simulink model "two_level_sixphase_f_sw_counter"  (R2021a)
settings: Solver=FixedStepDiscrete  StartTime=0.0  StopTime=0.030  RelTol=1e-3
libraries: hdlsllib x1
settings Model: DataTypeOverride=Off  Creator=micha  LastModifiedBy=micha
settings SolverCC: AlgebraicLoopSolver=TrustRegion  AutoInsertRateTranBlk=on
settings DataIOCC: LimitDataPoints=on  SaveOutput=off  SaveTime=off
settings OptimizationCC: BlockReduction=off  ConditionallyExecuteInputs=off  DefaultParameterBehavior=Inlined  LifeSpan=inf
settings DebuggingCC: AlgebraicLoopMsg=error  SingleTaskRateTransMsg=error  AllowSymbolicDim=off  StrictBusMsg=ErrorOnBusTreatedAsVector  SFUnexpectedBacktrackingDiag=warning  SFNoUnconditionalDefaultTransitionDiag=warning  SFExecutionAtInitializationDiag=none  SFMachineParentedDataDiag=warning  ArithmeticOperatorsInVariantConditions=warning
settings HardwareCC: ProdBitPerPointer=32  ProdBitPerSizeT=32  ProdBitPerPtrDiffT=32  ProdLargestAtomicFloat=None  ProdIntDivRoundTo=Undefined  ProdEndianess=Unspecified  ProdWordSize=32  ProdHWDeviceType=ASIC/FPGA->ASIC/FPGA  ProdEqTarget=off
settings SFSimCC: SimUseLocalCustomCode=off  CustomCodeUndefinedFunction=UseInterfaceOnly
settings RTWCC: RTWUseLocalCustomCode=off
settings CodeAppCC: StateflowObjectComments=on
settings GRTTargetCC: TargetLangStandard=C89/C90 (ANSI)
settings ConfigComp: CovScope=ReferencedModels  CovMetricSettings=dw  CovSaveCumulativeToWorkspaceVar=on  CovSaveSingleToWorkspaceVar=on  CovExternalEMLEnable=off  CovSFcnEnable=off

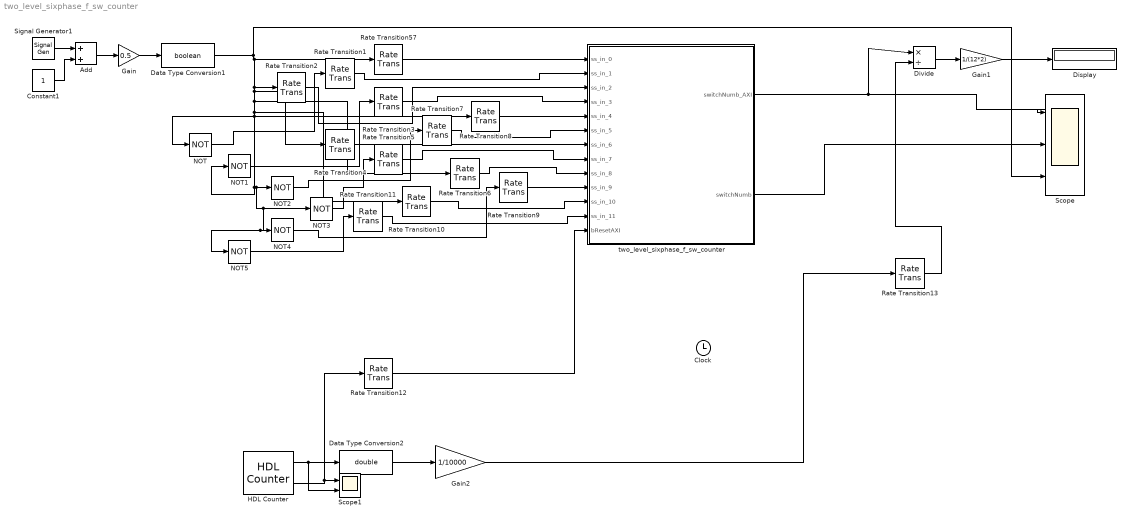
== system two_level_sixphase_f_sw_counter ==
  Add : Sum
  Clock : Clock
  Constant1 : Constant
  Data Type Conversion1 : DataTypeConversion  OutDataTypeStr=boolean
  Data Type Conversion2 : DataTypeConversion  OutDataTypeStr=double
  Display : Display
  Divide : Product  Inputs=*/
  Gain : Gain  Gain=0.5
  Gain1 : Gain  Gain=1/(12*2)
  Gain2 : Gain  Gain=1/10000
  HDL Counter : hdlsllib/Sources/HDL Counter  CountType=Count limited  CountInit=0  CountStep=1  CountMax=100  CountFromType=Initial value  CountFrom=0  CountResetPort=off  CountLoadPort=off  CountEnbPort=off  CountDirPort=off  CountHitOutputPort=on  CountDataType=Unsigned  CountWordLen=32  CountFracLen=0  CountSampTime=100e-6
  NOT{,1..5} (6 alike) : Logic  Operator=NOT  IconShape=distinctive  AllPortsSameDT=off  OutDataTypeStr=boolean
  Rate Transition{1..13,57} (14 alike) : RateTransition  OutPortSampleTime=t_clock
  Scope : Scope  NumInputPorts=3
  Scope1 : Scope  NumInputPorts=2
  Signal Generator1 : SignalGenerator  WaveForm=square  Frequency=2*pi*10000  Units=rad/sec
  two_level_sixphase_f_sw_counter : Subsystem  TreatAsAtomicUnit=on
  wires:
  Rate Transition57/1 -> two_level_sixphase_f_sw_counter/1(ss_in_0)
  Rate Transition1/1 -> two_level_sixphase_f_sw_counter/2(ss_in_1)
  Rate Transition2/1 -> two_level_sixphase_f_sw_counter/3(ss_in_2)
  Rate Transition3/1 -> two_level_sixphase_f_sw_counter/4(ss_in_3)
  Rate Transition4/1 -> two_level_sixphase_f_sw_counter/7(ss_in_6)
  Rate Transition5/1 -> two_level_sixphase_f_sw_counter/8(ss_in_7)
  Rate Transition6/1 -> two_level_sixphase_f_sw_counter/9(ss_in_8)
  Rate Transition7/1 -> two_level_sixphase_f_sw_counter/6(ss_in_5)
  Rate Transition8/1 -> two_level_sixphase_f_sw_counter/5(ss_in_4)
  Rate Transition9/1 -> two_level_sixphase_f_sw_counter/10(ss_in_9)
  Rate Transition10/1 -> two_level_sixphase_f_sw_counter/11(ss_in_10)
  Rate Transition11/1 -> two_level_sixphase_f_sw_counter/12(ss_in_11)
  HDL Counter/2 -> Scope1/1, Rate Transition12/1
  Rate Transition12/1 -> two_level_sixphase_f_sw_counter/13(bResetAXI)
  two_level_sixphase_f_sw_counter/1(switchNumb_AXI) -> Scope/1, Divide/1
  two_level_sixphase_f_sw_counter/2(switchNumb) -> Scope/2
  Add/1 -> Gain/1
  Signal Generator1/1 -> Add/1
  Constant1/1 -> Add/2
  Gain/1 -> Data Type Conversion1/1
  Data Type Conversion1/1 -> Rate Transition57/1, Rate Transition4/1, Rate Transition6/1, Rate Transition10/1, NOT5/1, NOT4/1, NOT3/1, NOT2/1, NOT1/1, NOT/1, Rate Transition8/1, Rate Transition2/1, Scope/3
  NOT/1 -> Rate Transition1/1
  NOT1/1 -> Rate Transition3/1
  NOT2/1 -> Rate Transition7/1
  NOT3/1 -> Rate Transition5/1
  NOT4/1 -> Rate Transition9/1
  NOT5/1 -> Rate Transition11/1
  Divide/1 -> Gain1/1
  Gain1/1 -> Display/1
  HDL Counter/1 -> Data Type Conversion2/1, Scope1/2
  Rate Transition13/1 -> Divide/2
  Gain2/1 -> Rate Transition13/1
  Data Type Conversion2/1 -> Gain2/1

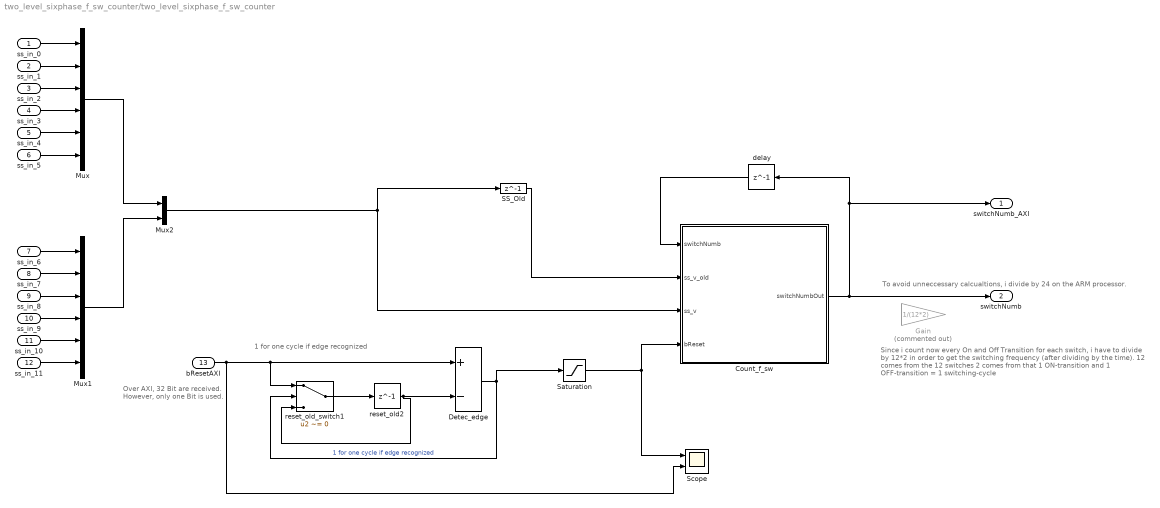
== system two_level_sixphase_f_sw_counter/two_level_sixphase_f_sw_counter ==
  note: To avoid unneccessary calcualtions, i divide by 24 on the ARM processor.
  note: 1 for one cycle if edge recognized
  note: Over AXI, 32 Bit are received.
      | However, only one Bit is used.
  note: Since i count now every On and Off Transition for each switch,
      |  i have to divide by 12*2 in order to get the switching frequency
      |  (after dividing by the time).
      | 12 comes from the 12 switches
      | 2 comes from that 1 ON-transition and 1 OFF-transition = 1 switching-cycle
  ss_in_0 : Inport
  ss_in_1 : Inport  Port=2
  ss_in_2 : Inport  Port=3
  ss_in_3 : Inport  Port=4
  ss_in_4 : Inport  Port=5
  ss_in_5 : Inport  Port=6
  ss_in_6 : Inport  Port=7
  ss_in_7 : Inport  Port=8
  ss_in_8 : Inport  Port=9
  ss_in_9 : Inport  Port=10
  ss_in_10 : Inport  Port=11
  ss_in_11 : Inport  Port=12
  bResetAXI : Inport  Port=13
  Count_f_sw : MATLAB Function  TreatAsAtomicUnit=on  VariantControl=(default)
  Detec_edge : Sum  Inputs=+-  AccumDataTypeStr=int8  OutDataTypeStr=int8
  Gain : Gain  Commented=on  Gain=1/(12*2)
  Mux : Mux  Inputs=6
  Mux1 : Mux  Inputs=6
  Mux2 : Mux  Inputs=2
  SS_Old : Delay  DelayLength=1
  Saturation : Saturate  UpperLimit=1  LowerLimit=0  OutMin=[0]  OutMax=[1]  OutDataTypeStr=fixdt(0,1)
  Scope : Scope  NumInputPorts=2
  delay : Delay  DelayLength=1
  reset_old2 : Delay  DelayLength=1
  reset_old_switch1 : Switch  Criteria=u2 ~= 0
  switchNumb_AXI : Outport  VectorParamsAs1DForOutWhenUnconnected=off
  switchNumb : Outport  Port=2  VectorParamsAs1DForOutWhenUnconnected=off
  wires:
  Count_f_sw/1(switchNumbOut) -> delay/1, switchNumb_AXI/1, switchNumb/1
  SS_Old/1 -> Count_f_sw/2(ss_v_old)
  Mux1/1 -> Mux2/2
  ss_in_3/1 -> Mux/4
  ss_in_0/1 -> Mux/1
  reset_old_switch1/1 -> reset_old2/1
  ss_in_11/1 -> Mux1/6
  Saturation/1 -> Count_f_sw/4(bReset), Scope/1
  ss_in_7/1 -> Mux1/2
  Mux2/1 -> SS_Old/1, Count_f_sw/3(ss_v)
  ss_in_5/1 -> Mux/6
  bResetAXI/1 -> Scope/2, reset_old_switch1/1, Detec_edge/1
  Detec_edge/1 -> Saturation/1, reset_old_switch1/2  "1 for one cycle if edge recognized"
  delay/1 -> Count_f_sw/1(switchNumb)
  ss_in_4/1 -> Mux/5
  Mux/1 -> Mux2/1
  ss_in_2/1 -> Mux/3
  ss_in_9/1 -> Mux1/4
  reset_old2/1 -> Detec_edge/2, reset_old_switch1/3
  ss_in_10/1 -> Mux1/5
  ss_in_1/1 -> Mux/2
  ss_in_8/1 -> Mux1/3
  ss_in_6/1 -> Mux1/1

== matlab function two_level_sixphase_f_sw_counter/Count_f_sw ==
  data: switchNumb input fixdt(0,25,0); ss_v_old input; ss_v input; switchNumbOut output fixdt(0,25,0); bReset input
 function switchNumbOut   = Count_f_sw(switchNumb,ss_v_old,ss_v, bReset)
   %
    %% toDO
        %s
 
    %% Initialization
    Fq25    = fimath('RoundingMethod', 'Floor', 'OverflowAction', 'Wrap','ProductMode', 'FullPrecision', 'ProductWordLength', 25,'ProductFractionLength',0,'SumMode','SpecifyPrecision','SumWordLength',25,'SumFractionLength',0);

    % I need this initialization, in order that the HDL Coder and Simulink knows the size of the vectors! Without these, i will get an error!
   % idx_globalOld     = fi(1, 0, 8, 0); % Chosen position overall in the error vector
    %switchNumb = fi(0, 0, 25, 0);
    
    %% Reset the counters (similar to the THD, i will try to average the switching frequency over 20 fundamental periods. After this time, a Reset-Flag from the ARM processor will reset the counter) 
    if (bReset == true) 
        switchNumb = fi(0, 0, 25, 0);
    end
    %% Check if switching occurs. If yes count up.
    % However, dependent of the ss_v before, switching can but do not have to occure, if the previously applied ss_v keeps.

    %Use a for-loop since in VHDL i have time and can do a resource streaming
    %Even if i need 6 cycles @100MHz, since it is not able to have have
    %switching (on/off inside of 60ns), this is ok (because T_cf = 10us and
    %and switching for such a short time is not allwoed nayway, since it is
    %not worth it (too much losses).)
    for countSS=fi(1, 0, 8, 0):fi(12, 0, 8, 0) %1:12
        if (ss_v(countSS) ~= ss_v_old(countSS)) %Check if switch has changed
            switchNumb = fi(add(Fq25,switchNumb,fi(1, 0, 25, 0)),0,25,0); % +1 Increment the switch counter +1
        end
    end

    switchNumbOut = switchNumb;

 end
